simulink model "two_link_planar_manipulator"  (R2023a)
settings: Solver=VariableStepAuto  StartTime=0.0  StopTime=10.0  RelTol=1e-3
values from neighbouring files (symbols this model uses):
  K = lqr(A,B,Q,R)    [two_link_planar_manipulator_sim.m]
libraries: robotmaniplib x1, simulink x1
settings Model: Creator=donelanp  LastModifiedBy=donelanp

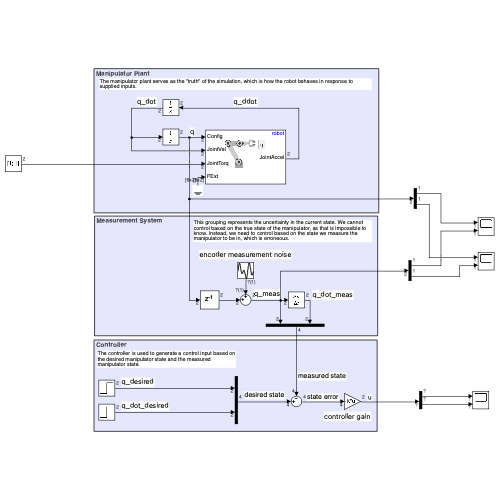
[thumbnail: Simulink's stored preview of the top-level diagram]
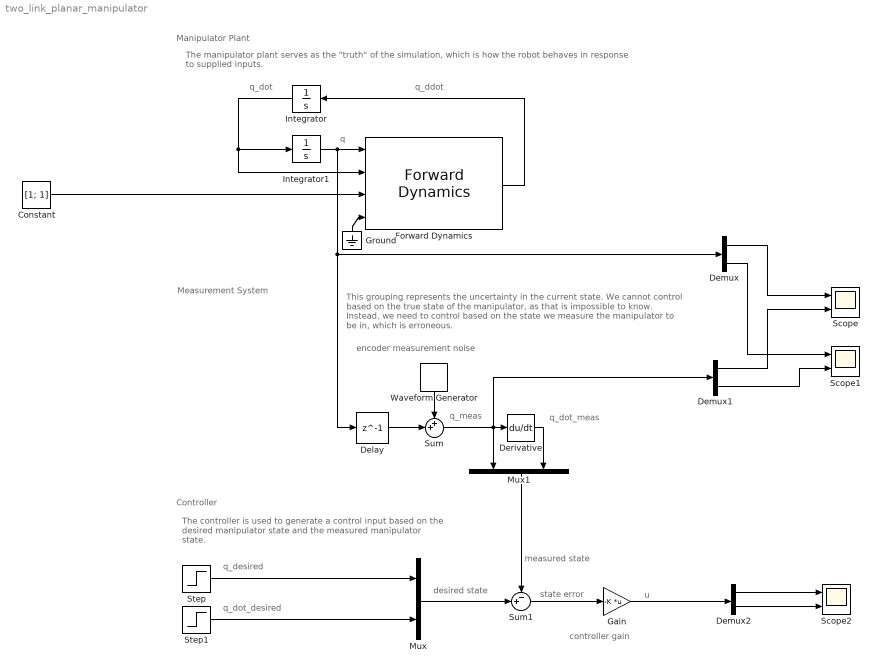
== system two_link_planar_manipulator ==
  note: This grouping represents the uncertainty in the current state. We cannot control based on the true state of the manipulator, as that is impossible to know. Instead, we need to control based on the state we measure the manipulator to be in, which is erroneous.
  note: The manipulator plant serves as the "truth" of the simulation, which is how the robot behaves in response to supplied inputs.
  note: u
  note: Controller
  note: desired state
  note: state error
  note: controller gain
  note: q_desired
  note: q_dot_meas
  note: Measurement System
  note: encoder measurement noise
  note: q_meas
  note: Manipulator Plant
  note: q
  note: q_dot
  note: q_ddot
  note: q_dot_desired
  note: measured state
  note: The controller is used to generate a control input based on the desired manipulator state and the measured manipulator state.
  Constant : Constant  Value=[1; 1]
  Delay : Delay  DelayLength=1
  Demux : Demux  Outputs=2
  Demux1 : Demux  Outputs=2
  Demux2 : Demux  Outputs=2
  Derivative : Derivative
  Forward Dynamics : robotmaniplib/Forward Dynamics  RigidBodyTree=robot  SimulateUsing=Interpreted execution
  Gain : Gain  Gain=-K  Multiplication=Matrix(K*u)
  Ground : Ground
  Integrator : Integrator  InitialCondition=[0;0]
  Integrator1 : Integrator  InitialCondition=[0;0]
  Mux : Mux  Inputs=2
  Mux1 : Mux  Inputs=2
  Scope : Scope  NumInputPorts=2
  Scope1 : Scope  NumInputPorts=2
  Scope2 : Scope  NumInputPorts=2
  Step : Step  Before=[0;0]  After=[1;1]  SampleTime=0
  Step1 : Step  Before=[0;0]  After=[1;1]  SampleTime=0
  Sum : Sum  Inputs=++|
  Sum1 : Sum  Inputs=-+|
  Waveform Generator : simulink/Sources/Waveform Generator  OutMin=[]  OutMax=[]  OutDataTypeStr=double  SelectedSignal=1  Signals=0  BlockNames=MultiportSwitch_882f284701a34e8  SampleTime=0.1
  wires:
  Forward Dynamics/1 -> Integrator/1
  Integrator/1 -> Forward Dynamics/2, Integrator1/1
  Integrator1/1 -> Demux/1, Delay/1, Forward Dynamics/1
  Delay/1 -> Sum/2
  Waveform Generator/1 -> Sum/1
  Sum/1 -> Demux1/1, Derivative/1, Mux1/1
  Ground/1 -> Forward Dynamics/4
  Step/1 -> Mux/1
  Step1/1 -> Mux/2
  Mux1/1 -> Sum1/1
  Mux/1 -> Sum1/2
  Sum1/1 -> Gain/1
  Gain/1 -> Demux2/1
  Constant/1 -> Forward Dynamics/3
  Derivative/1 -> Mux1/2
  Demux/1 -> Scope/1
  Demux1/1 -> Scope/2
  Demux/2 -> Scope1/1
  Demux1/2 -> Scope1/2
  Demux2/1 -> Scope2/1
  Demux2/2 -> Scope2/2
